simulink model "TopLevel_Turbofan_DT_PDM"  (R2025a)
settings: Solver=ode15s  StartTime=0.0  StopTime=500  MaxStep=0.01  RelTol=1e-3
undefined symbols (not defined in the file or in its folder): BPR_design, DoUpgrade, Eff_hpt_map, Eff_Mod_Fan, Eff_Mod_HPC, Eff_Mod_HPC_Up, Eff_Mod_HPT, Eff_Mod_HPT_Up, Eff_Mod_LPC, Eff_Mod_LPC_Up, Eff_Mod_LPT, eta_hpc_map, eta_lpc_map, eta_lpt_map, Fan_eta_data, Fan_PR_data, FaultMode, flow_vec_fan, norm_flow_hpt, norm_speed_hpt, PR_hpc_map, PR_lpc_map, PR_lpt_map, speed_vec_fan, speed_vec_hpc, speed_vec_lpc, speed_vec_lpt, Torque_hpt_map, Wc_hpc_bp, Wc_lpc_bp, Wc_lpt_bp
libraries: fl_lib x10, nesl_utility x10, simulink x2, sdl_lib x2
(part 2 of 2)

== matlab function TopLevel_Turbofan_DT_PDM/LPC/LPC_CoreCalc ==
  data: P2_in input; P3 output; T2_in input; PR_LPC input; eta_LPC input; N1_RPM input; Wc_core_in input; T3 output; Torque_LPC output; m_dot_core output
function [P3, T3, Torque_LPC, m_dot_core] = ...
    LPC_CoreCalc(P2_in, T2_in, PR_LPC, eta_LPC, N1_RPM, Wc_core_in)

% ===== constants & guards ==============================================
gamma = 1.4;  cp = 1004;  Tref = 288.15;  Pref = 101325;

P2 = max(P2_in,    1e-3);
T2 = max(T2_in,    1e-3);
PR = max(PR_LPC,   1.0);      % compressor PR ≥ 1
eta = max(eta_LPC, 1e-3);
rpm = max(N1_RPM,  1e-3);
Wc  = max(Wc_core_in, 1e-3);

% ===== outlet P/T =======================================================
P3 = P2 * PR;
T3 = T2 * (1 + (1/eta)*(PR^((gamma-1)/gamma) - 1));

% ===== mass-flow recovery (real kg/s) ===================================
temp_ratio  = max(T2 / Tref, eps);
press_ratio = max(P2 / Pref, eps);
m_dot_core  = Wc * sqrt(temp_ratio) * press_ratio;

% ===== torque ===========================================================
omega  = max(rpm * 2*pi/60, eps);
delta_h = cp * max(T3 - T2, 0);
torque_raw = (m_dot_core * delta_h) / omega;
Torque_LPC = min(max(torque_raw, -1e6), 1e6);
end

== matlab function TopLevel_Turbofan_DT_PDM/HPT/ComputeTorqueFinal ==
  data: thermoTorque input; Torque_HPT output; mapTorque input
function Torque_HPT = ComputeTorqueFinal(thermoTorque, mapTorque)
    % Combine both torque calculations with 50/50 weighting
    Torque_HPT = 0.5 * thermoTorque + 0.5 * mapTorque;
end

== matlab function TopLevel_Turbofan_DT_PDM/HPT/HPT_TempCalc ==
  data: P5_in input; P6_out output; T5_in input; Eff_HPT input; T6_out output
function [P6_out, T6_out] = HPT_TempCalc(P5_in, T5_in, Eff_HPT)
    gamma = 1.33;
    PR_turb = 1.0;  % Assume isobaric turbine
    T6_ideal = T5_in * (PR_turb)^((gamma-1)/gamma);
    T6_out = T5_in - Eff_HPT * (T5_in - T6_ideal);
    P6_out = P5_in;  % no pressure drop assumption
end

== matlab function TopLevel_Turbofan_DT_PDM/HPT/HPT_TorqueCalc ==
  data: m_dot5 input; Torque_HPT output; T5_in input; T6_out input; omega_N2 input
function Torque_HPT = HPT_TorqueCalc(m_dot5, T5_in, T6_out, omega_N2)
    cp = 1150;  % J/kg-K
    work = cp * (T5_in - T6_out);

    % Safety wrappers
    omega_safe = max(omega_N2, eps);
    m_dot_safe = max(m_dot5, eps);      % protect m_dot
    work_safe = max(work, 0);           % assume zero torque if temp reversed

    Torque_HPT = (m_dot_safe * work_safe) / omega_safe;
end
